simulink model "Modelo_LeyDeControlMinima_Complementaria"  (R2026a)
settings: Solver=VariableStepAuto
values from neighbouring files (symbols this model uses):
  alpha_Cu = 3.9e-3    (= 0.0039)    [coeficientes.m]
  b_eq = b_m + b_l/(r_m2l^2)    (= 2.19444444444e-05)    [coeficientes.m]
  C_ts = 0.818    [coeficientes.m]
  g = 9.80665    [coeficientes.m]
  J_eq = J_m + J_l/(r_m2l^2)    (= 4.58263888889e-05)    [coeficientes.m]
  k_l = 0.1    [coeficientes.m]
  L_d = 6.6e-3    (= 0.0066)    [coeficientes.m]
  L_ls = 0.8e-3    (= 0.0008)    [coeficientes.m]
  L_q = 5.8e-3    (= 0.0058)    [coeficientes.m]
  lambda = 0.016    [coeficientes.m]
  Pp = 3    [coeficientes.m]
  r_m2l = 120.0    (= 120)    [coeficientes.m]
  R_sREF = 1.02    [coeficientes.m]
  R_tsamb = 146.7    [coeficientes.m]
  T_amb = 20    [coeficientes.m]
  T_sREF = 20    [coeficientes.m]
libraries: eeTransforms x5
settings Model: Creator=barrios14101  LastModifiedBy=admin

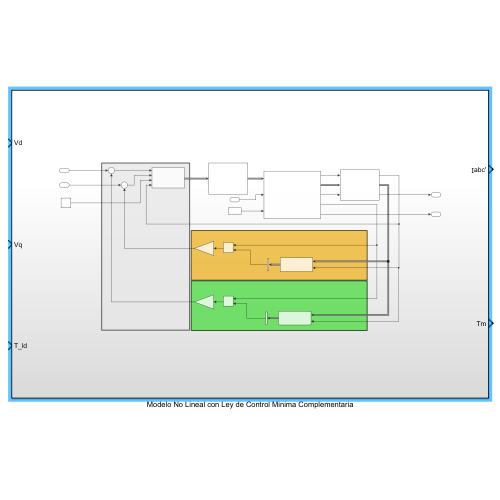
[thumbnail: Simulink's stored preview of the top-level diagram]
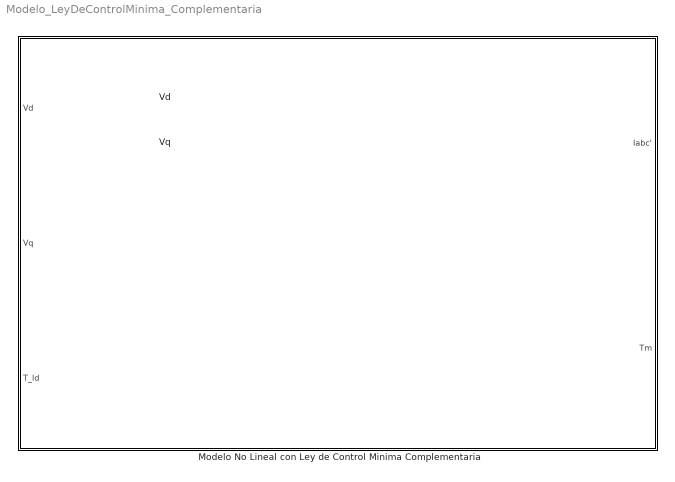
== system Modelo_LeyDeControlMinima_Complementaria ==
  Vq : Inport
  Vd : Inport  Port=2
  Modelo No Lineal con Ley de Control Minima Complementaria : Subsystem

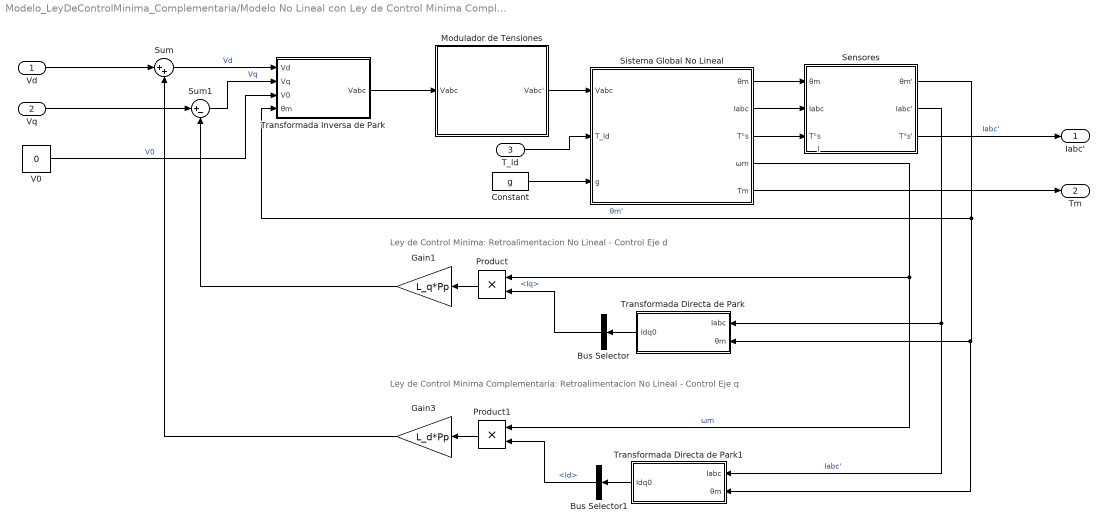
== system Modelo_LeyDeControlMinima_Complementaria/Modelo No Lineal con Ley de Control Minima Complementaria ==
  note: Ley de Control Minima: Retroalimentacion No Lineal - Control Eje d
  note: Ley de Control Minima Complementaria: Retroalimentacion No Lineal - Control Eje q
  note: Ⅰ
  Vd : Inport
  Vq : Inport  Port=2
  T_ld : Inport  Port=3
  Bus Selector : BusSelector  OutputSignals=Ⅰq
  Bus Selector1 : BusSelector  OutputSignals=Ⅰd
  Constant : Constant  Value=g
  Gain1 : Gain  Gain=L_q*Pp
  Gain3 : Gain  Gain=L_d*Pp
  Modulador de Tensiones : Subsystem
  Product : Product
  Product1 : Product
  Sensores : Subsystem
  Sistema Global No Lineal : Subsystem
  Sum : Sum  Inputs=|++
  Sum1 : Sum  Inputs=|+-
  Transformada Directa de Park : Subsystem
  Transformada Directa de Park1 : Subsystem
  Transformada Inversa de Park : Subsystem
  V0 : Constant  Value=0
  Ⅰabc' : Outport
  Tm : Outport  Port=2
  wires:
  Gain3/1 -> Sum/2
  Product/1 -> Gain1/1
  Sensores/1(θm') -> Transformada Inversa de Park/4(θm), Transformada Directa de Park1/2(θm), Transformada Directa de Park/2(θm)  "θm'"
  Product1/1 -> Gain3/1
  Sensores/2(Ⅰabc') -> Transformada Directa de Park1/1(Ⅰabc), Transformada Directa de Park/1(Ⅰabc)  "Ⅰabc'"
  V0/1 -> Transformada Inversa de Park/3(V0)  "V0"
  Transformada Directa de Park1/1(Ⅰdq0) -> Bus Selector1/1
  Vd/1 -> Sum/1
  Bus Selector1/1 -> Product1/2  "<Ⅰd>"
  Gain1/1 -> Sum1/2
  T_ld/1 -> Sistema Global No Lineal/2(T_ld)
  Sistema Global No Lineal/4(ωm) -> Product1/1, Product/1  "ωm"
  Sum/1 -> Transformada Inversa de Park/1(Vd)  "Vd"
  Transformada Directa de Park/1(Ⅰdq0) -> Bus Selector/1
  Transformada Inversa de Park/1(Vabc) -> Modulador de Tensiones/1(Vabc)
  Sum1/1 -> Transformada Inversa de Park/2(Vq)  "Vq"
  Vq/1 -> Sum1/1
  Bus Selector/1 -> Product/2  "<Ⅰq>"
  Sistema Global No Lineal/5(Tm) -> Tm/1
  Sistema Global No Lineal/2(Ⅰabc) -> Sensores/2(Ⅰabc)
  Sistema Global No Lineal/1(θm) -> Sensores/1(θm)
  Sistema Global No Lineal/3(T°s) -> Sensores/3(T°s)
  Modulador de Tensiones/1(Vabc') -> Sistema Global No Lineal/1(Vabc)
  Constant/1 -> Sistema Global No Lineal/3(g)
  Sensores/3(T°s') -> Ⅰabc'/1  "Ⅰabc'"

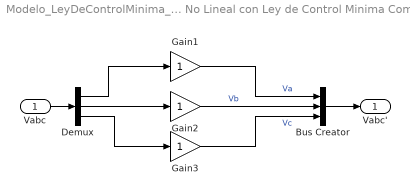
== system Modelo_LeyDeControlMinima_Complementaria/Modelo No Lineal con Ley de Control Minima Complementaria/Modulador de Tensiones ==
  Vabc : Inport
  Bus Creator : BusCreator  Inputs=3
  Demux : Demux  Outputs=3
  Gain1 : Gain
  Gain2 : Gain
  Gain3 : Gain
  Vabc' : Outport
  wires:
  Gain2/1 -> Bus Creator/2  "Vb"
  Gain3/1 -> Bus Creator/3  "Vc"
  Gain1/1 -> Bus Creator/1  "Va"
  Demux/2 -> Gain2/1
  Vabc/1 -> Demux/1
  Demux/1 -> Gain1/1
  Demux/3 -> Gain3/1
  Bus Creator/1 -> Vabc'/1

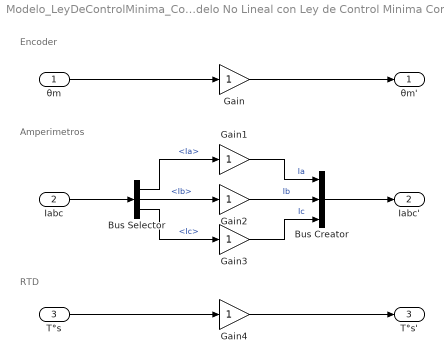
== system Modelo_LeyDeControlMinima_Complementaria/Modelo No Lineal con Ley de Control Minima Complementaria/Sensores ==
  note: Encoder
  note: Amperimetros
  note: RTD
  θm : Inport
  Ⅰabc : Inport  Port=2
  T°s : Inport  Port=3
  Bus Creator : BusCreator  Inputs=3
  Bus Selector : BusSelector  OutputSignals=Ⅰa,Ⅰb,Ⅰc
  Gain{,1..4} (5 alike) : Gain
  θm' : Outport
  Ⅰabc' : Outport  Port=2
  T°s' : Outport  Port=3
  wires:
  θm/1 -> Gain/1
  Gain/1 -> θm'/1
  T°s/1 -> Gain4/1
  Gain4/1 -> T°s'/1
  Bus Creator/1 -> Ⅰabc'/1
  Ⅰabc/1 -> Bus Selector/1
  Bus Selector/1 -> Gain1/1  "<Ⅰa>"
  Bus Selector/2 -> Gain2/1  "<Ⅰb>"
  Bus Selector/3 -> Gain3/1  "<Ⅰc>"
  Gain2/1 -> Bus Creator/2  "Ⅰb"
  Gain1/1 -> Bus Creator/1  "Ⅰa"
  Gain3/1 -> Bus Creator/3  "Ⅰc"

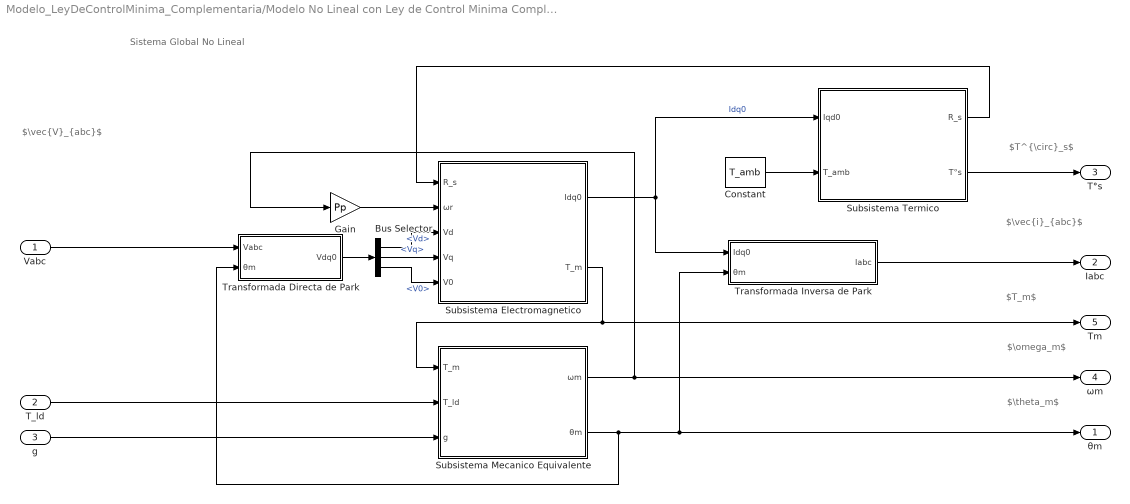
== system Modelo_LeyDeControlMinima_Complementaria/Modelo No Lineal con Ley de Control Minima Complementaria/Sistema Global No Lineal ==
  note: $\omega_m$
  note: $T^{\circ}_s$
  note: $\vec{i}_{abc}$
  note: $\vec{V}_{abc}$
  note: Sistema Global No Lineal
  note: $\theta_m$
  note: $T_m$
  Vabc : Inport
  T_ld : Inport  Port=2
  g : Inport  Port=3
  Bus Selector : BusSelector  OutputSignals=Vd,Vq,V0
  Constant : Constant  Value=T_amb
  Gain : Gain  Gain=Pp
  Subsistema Electromagnetico : Subsystem
  Subsistema Mecanico Equivalente : Subsystem
  Subsistema Termico : Subsystem
  Transformada Directa de Park : Subsystem
  Transformada Inversa de Park : Subsystem
  θm : Outport
  Ⅰabc : Outport  Port=2
  T°s : Outport  Port=3
  ωm : Outport  Port=4
  Tm : Outport  Port=5
  wires:
  Subsistema Termico/2(T°s) -> T°s/1
  Subsistema Electromagnetico/1(Ⅰdq0) -> Transformada Inversa de Park/1(Ⅰdq0), Subsistema Termico/1(Ⅰqd0)  "Ⅰdq0"
  Subsistema Mecanico Equivalente/1(ωm) -> Gain/1, ωm/1
  Subsistema Mecanico Equivalente/2(θm) -> Transformada Directa de Park/2(θm), Transformada Inversa de Park/2(θm), θm/1
  Subsistema Electromagnetico/2(T_m) -> Subsistema Mecanico Equivalente/1(T_m), Tm/1
  Subsistema Termico/1(R_s) -> Subsistema Electromagnetico/1(R_s)
  Gain/1 -> Subsistema Electromagnetico/2(ωr)
  T_ld/1 -> Subsistema Mecanico Equivalente/2(T_ld)
  Vabc/1 -> Transformada Directa de Park/1(Vabc)
  Constant/1 -> Subsistema Termico/2(T_amb)
  g/1 -> Subsistema Mecanico Equivalente/3(g)
  Transformada Directa de Park/1(Vdq0) -> Bus Selector/1
  Bus Selector/1 -> Subsistema Electromagnetico/3(Vd)  "<Vd>"
  Bus Selector/2 -> Subsistema Electromagnetico/4(Vq)  "<Vq>"
  Bus Selector/3 -> Subsistema Electromagnetico/5(V0)  "<V0>"
  Transformada Inversa de Park/1(Ⅰabc) -> Ⅰabc/1

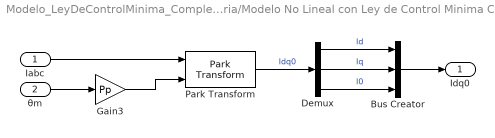
== system Modelo_LeyDeControlMinima_Complementaria/Modelo No Lineal con Ley de Control Minima Complementaria/Transformada Directa de Park ==
  Ⅰabc : Inport
  θm : Inport  Port=2
  Bus Creator : BusCreator  Inputs=3
  Demux : Demux  Outputs=3
  Gain3 : Gain  Gain=Pp
  Park Transform : eeTransforms/Park Transform  AxisAlignment=Q-axis  PowerInvariant=off
      settings: LibrarySourceBlock=|
      | ee_sl_lib/Mathematical
      | Transforms/Park Transform
  Ⅰdq0 : Outport
  wires:
  Gain3/1 -> Park Transform/2
  Park Transform/1 -> Demux/1  "Ⅰdq0"
  Demux/1 -> Bus Creator/1  "Ⅰd"
  Demux/3 -> Bus Creator/3  "Ⅰ0"
  Demux/2 -> Bus Creator/2  "Ⅰq"
  Bus Creator/1 -> Ⅰdq0/1
  Ⅰabc/1 -> Park Transform/1
  θm/1 -> Gain3/1

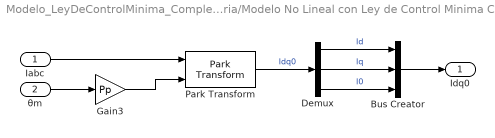
== system Modelo_LeyDeControlMinima_Complementaria/Modelo No Lineal con Ley de Control Minima Complementaria/Transformada Directa de Park1 ==
  Ⅰabc : Inport
  θm : Inport  Port=2
  Bus Creator : BusCreator  Inputs=3
  Demux : Demux  Outputs=3
  Gain3 : Gain  Gain=Pp
  Park Transform : eeTransforms/Park Transform  AxisAlignment=Q-axis  PowerInvariant=off
      settings: LibrarySourceBlock=|
      | ee_sl_lib/Mathematical
      | Transforms/Park Transform
  Ⅰdq0 : Outport
  wires:
  Gain3/1 -> Park Transform/2
  Park Transform/1 -> Demux/1  "Ⅰdq0"
  Demux/1 -> Bus Creator/1  "Ⅰd"
  Demux/3 -> Bus Creator/3  "Ⅰ0"
  Demux/2 -> Bus Creator/2  "Ⅰq"
  Bus Creator/1 -> Ⅰdq0/1
  Ⅰabc/1 -> Park Transform/1
  θm/1 -> Gain3/1

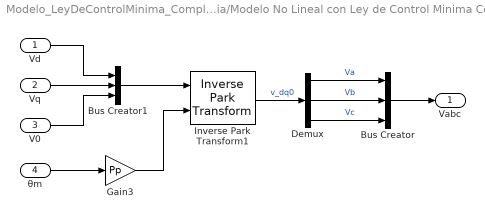
== system Modelo_LeyDeControlMinima_Complementaria/Modelo No Lineal con Ley de Control Minima Complementaria/Transformada Inversa de Park ==
  Vd : Inport
  Vq : Inport  Port=2
  V0 : Inport  Port=3
  θm : Inport  Port=4
  Bus Creator : BusCreator  Inputs=3
  Bus Creator1 : BusCreator  Inputs=3
  Demux : Demux  Outputs=3
  Gain3 : Gain  Gain=Pp
  Inverse Park Transform1 : eeTransforms/Inverse Park Transform  AxisAlignment=Q-axis  PowerInvariant=off
      settings: LibrarySourceBlock=|
      | ee_sl_lib/Mathematical
      | Transforms/Inverse
      | Park Transform
  Vabc : Outport
  wires:
  Gain3/1 -> Inverse Park Transform1/2
  Inverse Park Transform1/1 -> Demux/1  "v_dq0"
  Demux/1 -> Bus Creator/1  "Va"
  Demux/3 -> Bus Creator/3  "Vc"
  Demux/2 -> Bus Creator/2  "Vb"
  Bus Creator/1 -> Vabc/1
  θm/1 -> Gain3/1
  Vd/1 -> Bus Creator1/1
  Vq/1 -> Bus Creator1/2
  V0/1 -> Bus Creator1/3
  Bus Creator1/1 -> Inverse Park Transform1/1

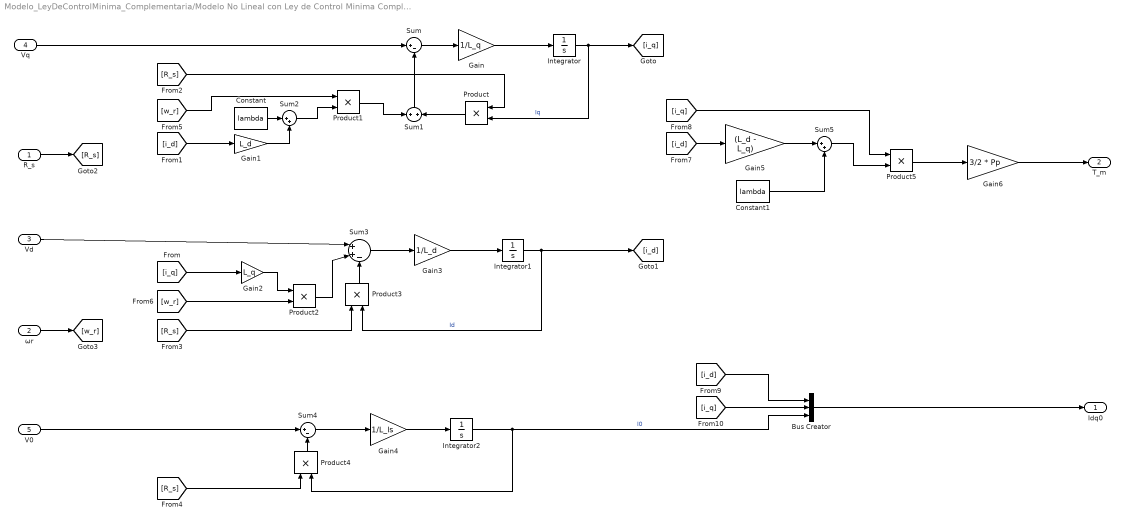
== system Modelo_LeyDeControlMinima_Complementaria/Modelo No Lineal con Ley de Control Minima Complementaria/Sistema Global No Lineal/Subsistema Electromagnetico ==
  R_s : Inport
  ωr : Inport  Port=2
  Vd : Inport  Port=3
  Vq : Inport  Port=4
  V0 : Inport  Port=5
  Bus Creator : BusCreator  Inputs=3
  Constant : Constant  Value=lambda
  Constant1 : Constant  Value=lambda
  Gain : Gain  Gain=1/L_q
  Gain1 : Gain  Gain=L_d
  Gain2 : Gain  Gain=L_q
  Gain3 : Gain  Gain=1/L_d
  Gain4 : Gain  Gain=1/L_ls
  Gain5 : Gain  Gain=(L_d - L_q)
  Gain6 : Gain  Gain=3/2 * Pp
  Integrator : Integrator
  Integrator1 : Integrator
  Integrator2 : Integrator
  Product{,1..5} (6 alike) : Product
  Sum : Sum  Inputs=|+-
  Sum1 : Sum
  Sum2 : Sum  Inputs=|++
  Sum3 : Sum  Inputs=|++-
  Sum4 : Sum  Inputs=|+-
  Sum5 : Sum  Inputs=|++
  Ⅰdq0 : Outport
  T_m : Outport  Port=2
  wires:
  Gain1/1 -> Sum2/2
  Product1/1 -> Sum1/1
  Sum2/1 -> Product1/2
  Constant/1 -> Sum2/1
  Product/1 -> Sum1/2
  Sum/1 -> Gain/1
  Sum1/1 -> Sum/2
  Vq/1 -> Sum/1
  Gain/1 -> Integrator/1
  Product3/1 -> Sum3/3
  Gain3/1 -> Integrator1/1
  Sum3/1 -> Gain3/1
  Product2/1 -> Sum3/2
  Gain2/1 -> Product2/1
  Vd/1 -> Sum3/1
  Product4/1 -> Sum4/2
  Integrator2/1 -> Bus Creator/3, Product4/2  "Ⅰ0"
  Gain4/1 -> Integrator2/1
  Sum4/1 -> Gain4/1
  V0/1 -> Sum4/1
  Gain5/1 -> Sum5/1
  Sum5/1 -> Product5/2
  Integrator1/1 -> [i_d], Product3/2  "Ⅰd"
  Constant1/1 -> Sum5/2
  Product5/1 -> Gain6/1
  Integrator/1 -> Product/2, [i_q]  "Ⅰq"
  Gain6/1 -> T_m/1
  [i_q] -> Gain2/1
  [i_d] -> Gain1/1
  [R_s] -> Product/1
  R_s/1 -> [R_s]
  [R_s] -> Product3/1
  [R_s] -> Product4/1
  ωr/1 -> [w_r]
  [w_r] -> Product1/1
  [w_r] -> Product2/2
  [i_d] -> Gain5/1
  [i_q] -> Product5/1
  [i_q] -> Bus Creator/2
  [i_d] -> Bus Creator/1
  Bus Creator/1 -> Ⅰdq0/1

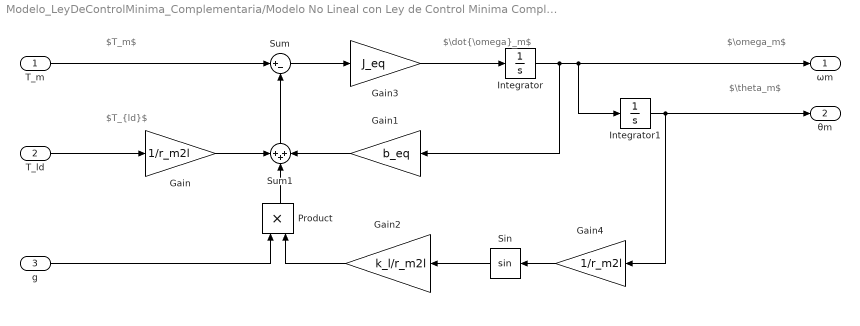
== system Modelo_LeyDeControlMinima_Complementaria/Modelo No Lineal con Ley de Control Minima Complementaria/Sistema Global No Lineal/Subsistema Mecanico Equivalente ==
  note: $T_m$
  note: $T_{ld}$
  note: $\dot{\omega}_m$
  note: $\omega_m$
  note: $\theta_m$
  T_m : Inport
  T_ld : Inport  Port=2
  g : Inport  Port=3
  Gain : Gain  Gain=1/r_m2l
  Gain1 : Gain  Gain=b_eq
  Gain2 : Gain  Gain=k_l/r_m2l
  Gain3 : Gain  Gain=J_eq
  Gain4 : Gain  Gain=1/r_m2l
  Integrator : Integrator
  Integrator1 : Integrator
  Product : Product
  Sin : Trigonometry
  Sum : Sum  Inputs=|+-
  Sum1 : Sum  Inputs=+++
  ωm : Outport
  θm : Outport  Port=2
  wires:
  Integrator/1 -> Integrator1/1, ωm/1, Gain1/1
  Integrator1/1 -> θm/1, Gain4/1
  Sum/1 -> Gain3/1
  T_m/1 -> Sum/1
  Sum1/1 -> Sum/2
  Gain2/1 -> Product/2
  Gain/1 -> Sum1/1
  Sin/1 -> Gain2/1
  Gain1/1 -> Sum1/3
  Gain3/1 -> Integrator/1
  Gain4/1 -> Sin/1
  T_ld/1 -> Gain/1
  Product/1 -> Sum1/2
  g/1 -> Product/1

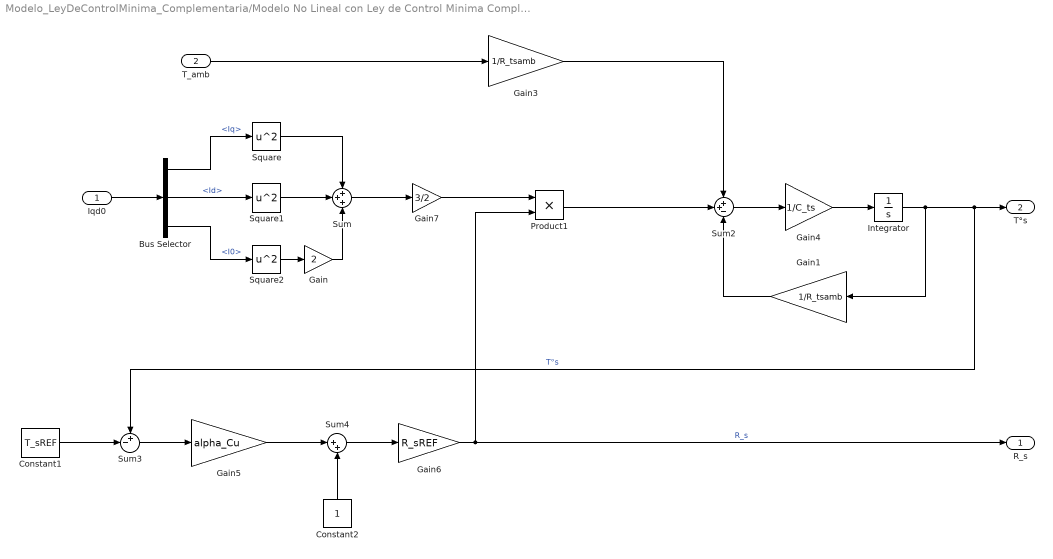
== system Modelo_LeyDeControlMinima_Complementaria/Modelo No Lineal con Ley de Control Minima Complementaria/Sistema Global No Lineal/Subsistema Termico ==
  Ⅰqd0 : Inport
  T_amb : Inport  Port=2
  Bus Selector : BusSelector  OutputSignals=Ⅰq,Ⅰd,Ⅰ0
  Constant1 : Constant  Value=T_sREF
  Constant2 : Constant
  Gain : Gain  Gain=2
  Gain1 : Gain  Gain=1/R_tsamb
  Gain3 : Gain  Gain=1/R_tsamb
  Gain4 : Gain  Gain=1/C_ts
  Gain5 : Gain  Gain=alpha_Cu
  Gain6 : Gain  Gain=R_sREF
  Gain7 : Gain  Gain=3/2
  Integrator : Integrator
  Product1 : Product
  Square : Math  Operator=square
  Square1 : Math  Operator=square
  Square2 : Math  Operator=square
  Sum : Sum  Inputs=+++
  Sum2 : Sum  Inputs=++-
  Sum3 : Sum  Inputs=+-|
  Sum4 : Sum  Inputs=|++
  R_s : Outport
  T°s : Outport  Port=2
  wires:
  Integrator/1 -> Gain1/1, Sum3/1, T°s/1  "T°s"
  Gain6/1 -> R_s/1, Product1/2  "R_s"
  Gain7/1 -> Product1/1
  Sum4/1 -> Gain6/1
  Constant1/1 -> Sum3/2
  Gain/1 -> Sum/3
  Gain5/1 -> Sum4/1
  Sum3/1 -> Gain5/1
  T_amb/1 -> Gain3/1
  Sum/1 -> Gain7/1
  Constant2/1 -> Sum4/2
  Square2/1 -> Gain/1
  Sum2/1 -> Gain4/1
  Square1/1 -> Sum/2
  Square/1 -> Sum/1
  Product1/1 -> Sum2/2
  Gain4/1 -> Integrator/1
  Gain1/1 -> Sum2/3
  Gain3/1 -> Sum2/1
  Ⅰqd0/1 -> Bus Selector/1
  Bus Selector/2 -> Square1/1  "<Ⅰd>"
  Bus Selector/3 -> Square2/1  "<Ⅰ0>"
  Bus Selector/1 -> Square/1  "<Ⅰq>"

== system Modelo_LeyDeControlMinima_Complementaria/Modelo No Lineal con Ley de Control Minima Complementaria/Sistema Global No Lineal/Transformada Directa de Park ==
  Vabc : Inport
  θm : Inport  Port=2
  Bus Creator : BusCreator  Inputs=3
  Demux : Demux  Outputs=3
  Gain3 : Gain  Gain=Pp
  Park Transform : eeTransforms/Park Transform  AxisAlignment=Q-axis  PowerInvariant=off
      settings: LibrarySourceBlock=|
      | ee_sl_lib/Mathematical
      | Transforms/Park Transform
  Vdq0 : Outport
  wires:
  Gain3/1 -> Park Transform/2
  Park Transform/1 -> Demux/1  "v_dq0"
  Demux/1 -> Bus Creator/1  "Vd"
  Demux/3 -> Bus Creator/3  "V0"
  Demux/2 -> Bus Creator/2  "Vq"
  Bus Creator/1 -> Vdq0/1
  Vabc/1 -> Park Transform/1
  θm/1 -> Gain3/1

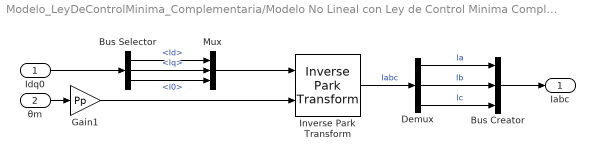
== system Modelo_LeyDeControlMinima_Complementaria/Modelo No Lineal con Ley de Control Minima Complementaria/Sistema Global No Lineal/Transformada Inversa de Park ==
  Ⅰdq0 : Inport
  θm : Inport  Port=2
  Bus Creator : BusCreator  Inputs=3
  Bus Selector : BusSelector  OutputSignals=Ⅰd,Ⅰq,Ⅰ0
  Demux : Demux  Outputs=3
  Gain1 : Gain  Gain=Pp
  Inverse Park Transform : eeTransforms/Inverse Park Transform  AxisAlignment=Q-axis  PowerInvariant=off
      settings: LibrarySourceBlock=|
      | ee_sl_lib/Mathematical
      | Transforms/Inverse
      | Park Transform
  Mux : Mux  Inputs=3
  Ⅰabc : Outport
  wires:
  Gain1/1 -> Inverse Park Transform/2
  Ⅰdq0/1 -> Bus Selector/1
  θm/1 -> Gain1/1
  Demux/1 -> Bus Creator/1  "Ⅰa"
  Inverse Park Transform/1 -> Demux/1  "Ⅰabc"
  Demux/2 -> Bus Creator/2  "Ⅰb"
  Bus Creator/1 -> Ⅰabc/1
  Demux/3 -> Bus Creator/3  "Ⅰc"
  Bus Selector/1 -> Mux/1  "<Ⅰd>"
  Bus Selector/2 -> Mux/2  "<Ⅰq>"
  Bus Selector/3 -> Mux/3  "<Ⅰ0>"
  Mux/1 -> Inverse Park Transform/1
